simulink model "FM_communication_system"  (Simulink 8.7)
settings: Solver=ode45  StartTime=0.0  StopTime=1  RelTol=1e-3
libraries: commanapbnd3 x2, commchan3 x1, dspfdesign x1, simulink_extras x1
settings Model: Creator=tp033402  LastModifiedBy=Muhammad Zubair
settings DataIOCC: SignalLoggingSaveFormat=ModelDataLogs
settings OptimizationCC: ExpressionDepthLimit=2147483647
settings DebuggingCC: SolverPrmCheckMsg=warning  FcnCallInpInsideContextMsg=UseLocalSettings  StateNameClashWarn=warning
settings GRTTargetCC: CombineOutputUpdateFcns=off  GRTInterface=on

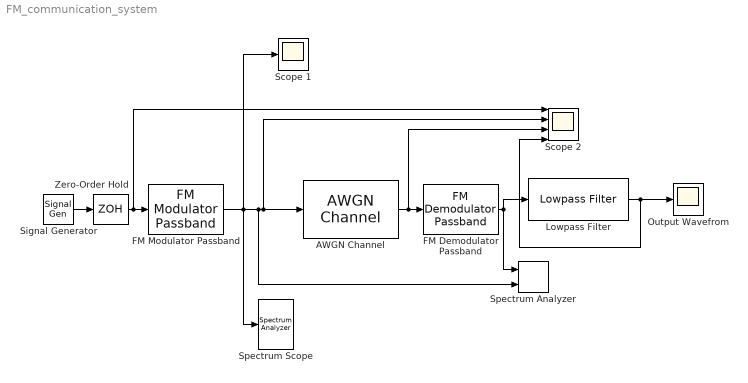
== system FM_communication_system ==
  AWGN Channel : commchan3/AWGN Channel  InputProcessing=Columns as channels (frame based)  seed=67  noiseMode="Signal to noise ratio  (SNR)"  EbNodB=10  EsNodB=10  SNRdB=50  bitsPerSym=1  Ps=1  Tsym=1  variance=1
  FM Demodulator Passband : commanapbnd3/FM Demodulator Passband  Fc=2000  Ph=0  Kc=1300  Ho=20
  FM Modulator Passband : commanapbnd3/FM Modulator Passband  Fc=2000  Ph=0  Kc=1300
  Lowpass Filter : dspfdesign/Lowpass Filter  FilterType=FIR  DesignForMinimumOrder=on  FilterOrder=50  PassbandFrequency=15.915  StopbandFrequency=2000  PassbandRipple=0.1  StopbandAttenuation=80  InheritSampleRate=off  SampleRate=44100  roundingMode=Floor  coeffsDataTypeStr=fixdt(1,16)  SimulateUsing=Interpreted execution
  Output Wavefrom : Scope
  Scope 1 : Scope
  Scope 2 : Scope  NumInputPorts=4
  Signal Generator : SignalGenerator  Frequency=100  Units=rad/sec
  Spectrum Analyzer : simulink_extras/Additional Sinks/Spectrum Analyzer  npts=1024  fftpts=1024  HowOften=128  sampleT=0.0001
  Spectrum Scope : SpectrumAnalyzer
  Zero-Order Hold : ZeroOrderHold  SampleTime=0.0001
  wires:
  FM Modulator Passband/1 -> Spectrum Analyzer/2, AWGN Channel/1, Scope 2/2, Spectrum Scope/1, Scope 1/1
  AWGN Channel/1 -> Scope 2/3, FM Demodulator Passband/1
  Signal Generator/1 -> Zero-Order Hold/1
  Zero-Order Hold/1 -> FM Modulator Passband/1, Scope 2/1
  FM Demodulator Passband/1 -> Lowpass Filter/1, Spectrum Analyzer/1
  Lowpass Filter/1 -> Scope 2/4, Output Wavefrom/1
